simulink model "Copy_of_PID"  (R2017a)
settings: Solver=ode5  StartTime=0.0  StopTime=30  FixedStep=0.05  MaxStep=0.05  RelTol=1e-3
libraries: simulink x2
settings Model: Creator=asus  LastModifiedBy=Lenovo

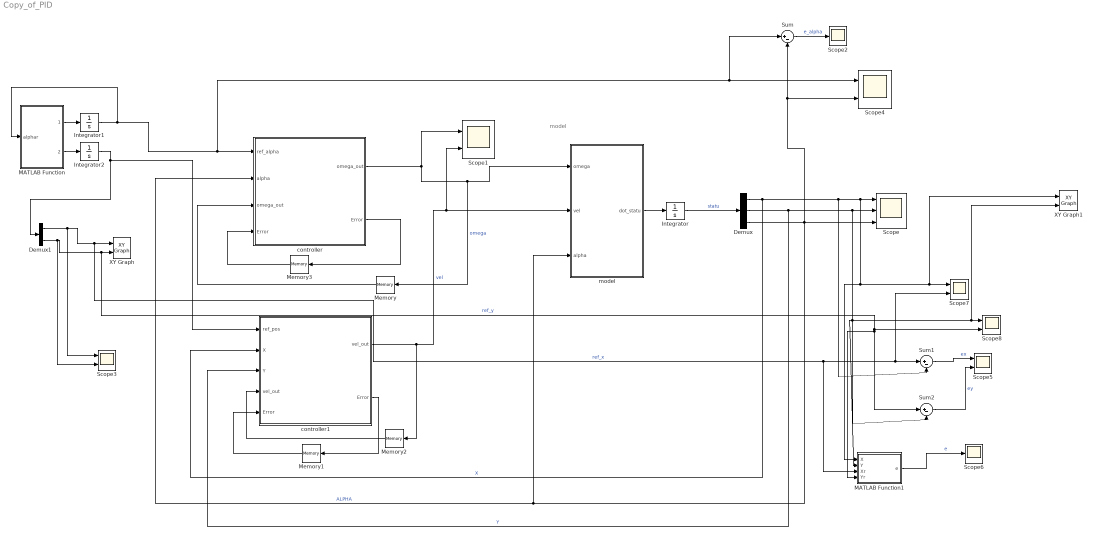
== system Copy_of_PID ==
  note: model
  Demux : Demux  Outputs=3
  Demux1 : Demux  Outputs=2
  Integrator : Integrator  InitialCondition=[1 -1 0 ]  IgnoreLimit=on
  Integrator1 : Integrator  InitialCondition=pi/3
  Integrator2 : Integrator
  MATLAB Function : MATLAB Function  TreatAsAtomicUnit=on
  MATLAB Function1 : MATLAB Function  TreatAsAtomicUnit=on
  Memory : Memory
  Memory1 : Memory  X0=[0 0 0 0]
  Memory2 : Memory
  Memory3 : Memory  X0=[0 0]
  Scope : Scope  NumInputPorts=3
  Scope{1,3..5,7..8} (6 alike) : Scope  NumInputPorts=2
  Scope2 : Scope
  Scope6 : Scope
  Sum : Sum  Inputs=|+-
  Sum1 : Sum  Inputs=|+-
  Sum2 : Sum  Inputs=|+-
  XY Graph : simulink/Sinks/XY Graph  xmin=-10  xmax=10  ymin=-10  ymax=10  st=-1
  XY Graph1 : simulink/Sinks/XY Graph  xmin=-10  xmax=10  ymin=-10  ymax=10  st=-1
  controller : MATLAB Function  TreatAsAtomicUnit=on
  controller1 : MATLAB Function  TreatAsAtomicUnit=on
  model : MATLAB Function  TreatAsAtomicUnit=on
  wires:
  Integrator/1 -> Demux/1  "statu"
  model/1(dot_statu) -> Integrator/1
  controller/1(omega_out) -> model/1(omega), Memory/1, Scope1/1  "omega"
  Memory/1 -> controller/3("omega_out ")
  controller/2(Error) -> Memory3/1
  Memory3/1 -> controller/4("Error ")
  MATLAB Function/1(dot_alphar) -> Integrator1/1
  Sum/1 -> Scope2/1  "e_alpha"
  controller1/1(vel_out) -> Memory2/1, Scope1/2, model/2(vel)  "vel"
  controller1/2(Error) -> Memory1/1
  Memory1/1 -> controller1/5("Error ")
  Demux/2 -> controller1/3(Y), MATLAB Function1/2(Y), XY Graph1/2, Scope8/1, Sum2/2, Scope/2  "Y"
  Demux/1 -> controller1/2(X), Sum1/2, XY Graph1/1, Scope7/1, MATLAB Function1/1(X), Scope/1  "X"
  MATLAB Function/2(dot_posr) -> Integrator2/1
  Demux/3 -> Scope4/2, Sum/2, model/3(alpha), controller/2(alpha), Scope/3  "ALPHA"
  Memory2/1 -> controller1/4("vel_out ")
  Demux1/1 -> Scope3/1, MATLAB Function1/3(Xr), Scope7/2, Sum1/1, XY Graph/1  "ref_x"
  Demux1/2 -> Scope3/2, Scope8/2, MATLAB Function1/4(Yr), Sum2/1, XY Graph/2  "ref_y"
  Integrator1/1 -> MATLAB Function/1(alphar), Sum/1, Scope4/1, controller/1(ref_alpha)
  Integrator2/1 -> Demux1/1, controller1/1(ref_pos)
  Sum1/1 -> Scope5/1  "ex"
  Sum2/1 -> Scope5/2  "ey"
  MATLAB Function1/1(e) -> Scope6/1  "e"

== matlab function Copy_of_PID/controller ==
  data: ref_alpha input; omega_out output; alpha input; omega_out input; Error input; Error output
function [omega_out,Error] = my_alpha_controller(ref_alpha, alpha, omega_out,Error)
% 程序上没有问题，在运动学模型上是可以完成任务的
% 最近修改时间：11. 20
% 基于运动学模型的   控制器
% u_out=[vx ;  omega]
% ref_vel=[xr yr alphar vr omegar]
% % e = [ex ey ealpha]
% 
% 

%% 状态量                                                                           
alpha = alpha;   alphar=ref_alpha;

e2k=alphar-alpha;

e2k_1=Error(1);
e2k_2=Error(2);


kp2=0.35;  ki2=0.02;  kd2=0.01;
delta_u2=kp2*(e2k-e2k_1)+ki2*e2k+kd2*(e2k-2*e2k_1+e2k_2);

omega_out=delta_u2+omega_out;

e2k_2=e2k_1;
e2k_1=e2k;

Error=[e2k_1;e2k_2];
end



































% %% 测试是否能得到
% %    statu=[2; -2; pi/2; 0.001; 0.001; 0.001];
% %    u_out=[0; 0];
% %    ref_pos=[0;0;pi/4]; ref_vel=[2; 0; 0];  
% %    Error=[0 0 0 0];
% %% 底盘参数
% % d = 0.18;	l = 0.16;	m = 24;	Iz = 11.89;	c = 513.6; %轮胎侧偏刚度
% 
% %% 状态量                                                                           
% x = statu(1);   y = statu(2);  alpha = statu(3); 
% vx = statu(4);  vy = statu(5);    omega = statu(6);
% 
% xr=ref_pos(1);  yr=ref_pos(2);  alphar=ref_pos(3);
% vxr=ref_vel(1); vyr=ref_vel(2); omegar=ref_vel(3);
% 
% % e1k_1=Error(1); e1k_2=Error(2);
% 
% e2k_1=Error(3); e2k_2=Error(4);
%                                                                                       
% %%  误差
% ex=x-xr;    ey=y-yr;    ealpha=alpha-alphar;
% ev=vx-vxr;  eomega=omega-omegar;
% 
% e1k=ex+ey;
% % kp1=  0.4  ;   ki1= 0.4   ;   kd1=  0.4  ;
% % delta_u1=kp1*(e1k-e1k_1)+ki1*e1k+kd1*(e1k-2*e1k_1+e1k_2);
% 
% e2k=ealpha;
% kp2=0.4;  ki2=0.4;  kd2=0.4;
% delta_u2=kp2*(e2k-e2k_1)+ki2*e2k+kd2*(e2k-2*e2k_1+e2k_2);
% 
% delta_uout=[delta_u1;delta_u2];
% 
% u_out = delta_uout+u_out;
% 
% e1k_2=e1k_1;
% e1k_1=e1k;
% 
% e2k_2=e2k_1;
% e2k_1=e2k;
% 
% Error=[e1k_1;   e1k_2;   e2k_1 ;   e2k_2];
% 
% 
%

== matlab function Copy_of_PID/model ==
  data: dot_statu output; omega input; vel input; alpha input
function dot_statu  = model(omega,vel,alpha)



dot_alpha = omega;
dot_X=vel*cos(alpha);
dot_Y=vel*sin(alpha);



% 状态【x y alpha vx vy omega】
dot_statu = [dot_X,dot_Y,dot_alpha];

end

% max=1/wheel_radius;
% for i=1:size(wheel_omega,2)
%     if wheel_omega(i)>max
%         wheel_omega(i) = max;
%     else
%         if wheel_omega(i)<-max
%             wheel_omega(i) = -max;
%         else
%             wheel_omega(i) = wheel_omega(i);
%         end
%     end
% end

== matlab function Copy_of_PID/MATLAB Function ==
  data: dot_alphar output; dot_posr output; alphar input
function [dot_alphar,dot_posr] = ref(alphar)


omegar=0;

velr=1;
dot_alphar = omegar;
dot_xr=velr*cos(alphar);
dot_yr=velr*sin(alphar);

dot_posr=[dot_xr;dot_yr];

end

== matlab function Copy_of_PID/controller1 ==
  data: ref_pos input; vel_out output; X input; Y input; vel_out input; Error input; Error output
function [vel_out,Error] = my_vel_controller(ref_pos, X,Y, vel_out,Error)
% 程序上没有问题，在运动学模型上是可以完成任务的
% 最近修改时间：11. 20
% 基于运动学模型的   控制器
% u_out=[vx ;  omega]
% ref_vel=[xr yr alphar vr omegar]
% % e = [ex ey ealpha]
% 
%
%% 状态量                                                                           
Xr =  ref_pos(1);   Yr =  ref_pos(2);
ex=Xr-X
ey=Yr-Y
%  ek=sqrt(ex^2+ey^2)        % 误差有问题
% rhor=sqrt(Xr^2+Yr^2);
% rho=sqrt(X^2+Y^2);
% e_rho=rhor-rho;
% aar=atan(Yr/Xr);
% aa=atan(Y/X);
% e_a=aar-aa;
% ek=e_rho+e_a;
ek=ex
ek_1=Error(1)
ek_2=Error(2)

ek1=ey
ek1_1=Error(3)
ek1_2=Error(4)

% kp=0.5;  ki=0.005;  kd=0.02;
% kp=0.4;  ki=0.0000001;  kd=0;
kpx=25;  kix=22;  kdx=0.2;
kpy=20;  kiy=0.05;  kdy=0;
delta_u=kpx*(ek-ek_1)+kix*ek+kdx*(ek-2*ek_1+ek_2)+...
    kpy*(ek1-ek1_1)+kiy*ek1+kdy*(ek1-2*ek1_1+ek1_2)

vel_out=delta_u+vel_out;

ek_2=ek_1;
ek_1=ek;

Error=[ek_1;ek_2;ek1_1;ek1_2];
end



































% %% 测试是否能得到
% %    statu=[2; -2; pi/2; 0.001; 0.001; 0.001];
% %    u_out=[0; 0];
% %    ref_pos=[0;0;pi/4]; ref_vel=[2; 0; 0];  
% %    Error=[0 0 0 0];
% %% 底盘参数
% % d = 0.18;	l = 0.16;	m = 24;	Iz = 11.89;	c = 513.6; %轮胎侧偏刚度
% 
% %% 状态量                                                                           
% x = statu(1);   y = statu(2);  alpha = statu(3); 
% vx = statu(4);  vy = statu(5);    omega = statu(6);
% 
% xr=ref_pos(1);  yr=ref_pos(2);  alphar=ref_pos(3);
% vxr=ref_vel(1); vyr=ref_vel(2); omegar=ref_vel(3);
% 
% % e1k_1=Error(1); e1k_2=Error(2);
% 
% e2k_1=Error(3); e2k_2=Error(4);
%                                                                                       
% %%  误差
% ex=x-xr;    ey=y-yr;    ealpha=alpha-alphar;
% ev=vx-vxr;  eomega=omega-omegar;
% 
% e1k=ex+ey;
% % kp1=  0.4  ;   ki1= 0.4   ;   kd1=  0.4  ;
% % delta_u1=kp1*(e1k-e1k_1)+ki1*e1k+kd1*(e1k-2*e1k_1+e1k_2);
% 
% e2k=ealpha;
% kp2=0.4;  ki2=0.4;  kd2=0.4;
% delta_u2=kp2*(e2k-e2k_1)+ki2*e2k+kd2*(e2k-2*e2k_1+e2k_2);
% 
% delta_uout=[delta_u1;delta_u2];
% 
% u_out = delta_uout+u_out;
% 
% e1k_2=e1k_1;
% e1k_1=e1k;
% 
% e2k_2=e2k_1;
% e2k_1=e2k;
% 
% Error=[e1k_1;   e1k_2;   e2k_1 ;   e2k_2];
% 
% 
%

== matlab function Copy_of_PID/MATLAB Function1 ==
  data: X input; e output; Y input; Xr input; Yr input
function e = fcn(X,Y,Xr,Yr)


rhor=sqrt(Xr^2+Yr^2);
rho=sqrt(X^2+Y^2);
e=rhor-rho


e= sqrt( (Yr-Y)^2  + (Xr-X)^2 )

end

% 42.4^2+42.4^2
% 
% 43.6^2+41.2^2
